simulink model "feedback_linearization_pp_HW_EKF"  (R2023a)
settings: Solver=FixedStepAuto  StartTime=0.0  StopTime=inf  FixedStep=0.001  RelTol=1e-3  EnableMultiTasking=on
values from neighbouring files (symbols this model uses):
  kpp = place(F,G,poles)    [Init_control.m]
  P = 0.5 * eye(6)    [Init_control.m]
undefined symbols (not defined in the file or in its folder): dev, lincontroller, Main, pwm_output0, quadParams
libraries: px4Sensorslib x2, px4lib x1
settings Model: SimulationMode=external  ExtModeTrigDuration=10  Creator=ArriGE66  LastModifiedBy=matte
settings SolverCC: PositivePriorityOrder=on
settings OptimizationCC: EnhancedBackFolding=on  PassReuseOutputArgsAs=Individual arguments  ZeroExternalMemoryAtStartup=off  ZeroInternalMemoryAtStartup=off  MaxStackSize=64  OptimizeBlockOrder=speed  DifferentSizesBufferReuse=on  EfficientTunableParamExpr=on
settings DebuggingCC: ParameterTunabilityLossMsg=error
settings HardwareCC: ProdBitPerPointer=32  ProdBitPerSizeT=32  ProdBitPerPtrDiffT=32  ProdLargestAtomicInteger=Long  ProdLargestAtomicFloat=Double  ProdWordSize=32  ProdLongLongMode=on  ProdHWDeviceType=ARM Compatible->ARM Cortex
settings SFSimCC: MATLABDynamicMemAlloc=off  SimTargetLang=C++
settings RTWCC: Description=Embedded Coder  SystemTargetFile=ert.tlc  HardwareBoard=PX4 Cube Orange  TemplateMakefile=ert_default_tmf  Toolchain=GNU Tools for PX4 Autopilots  TargetLang=C++
settings CodeAppCC: ForceParamTrailComments=on  IgnoreCustomStorageClasses=off  OperatorAnnotations=on  SimulinkDataObjDesc=on  SFDataObjDesc=on  InsertBlockDesc=on
settings ERTTargetCC: ExtMode=on  ExtModeTransport=3  ExtModeStaticAlloc=on  ExtModeStaticAllocSize=1024  ExtModeMexFile=ext_xcp  ExtModeMexArgs=1 COM10 3000000  ExtModeIntrfLevel=Level2 - Open

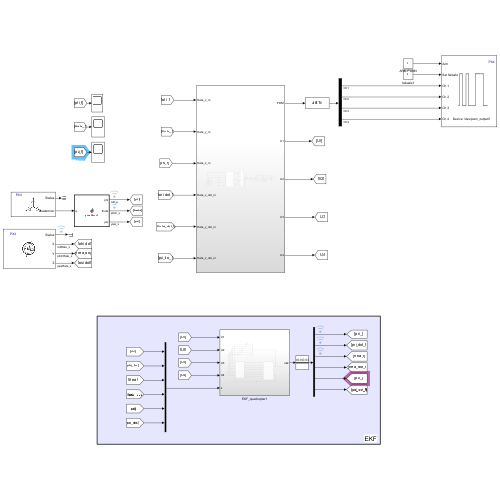
[thumbnail: Simulink's stored preview of the top-level diagram]
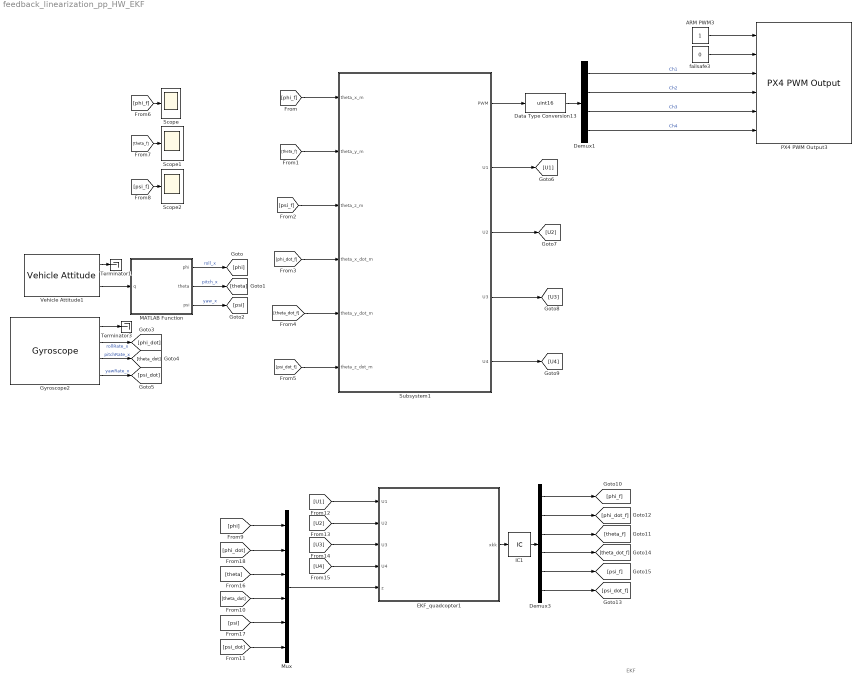
== system feedback_linearization_pp_HW_EKF ==
  note: EKF
  ARM PWM3 : Constant  OutDataTypeStr=boolean  SampleTime=0.002
  Data Type Conversion13 : DataTypeConversion  OutDataTypeStr=uint16  SaturateOnIntegerOverflow=off  RndMeth=Floor
  Demux1 : Demux
  Demux3 : Demux  Outputs=6
  EKF_quadcopter1 : Subsystem
  Gyroscope2 : px4Sensorslib/Gyroscope  uorbTimeStamp=off  BlockingMode=off  BlockTimeout=1e-3  sampleTime=0.002
  IC1 : InitialCondition  Value=[0;0;0;0;0;0]
  MATLAB Function : MATLAB Function  TreatAsAtomicUnit=on
  Mux : Mux  Inputs=6
  PX4 PWM Output3 : px4lib/PX4 PWM Output  pwmDevice=Main (/dev/pwm_output0)  pwmChannel1_=on  pwmChannel2_=on  pwmChannel3_=on  pwmChannel4_=on  pwmChannel5_=off  pwmChannel6_=off  pwmChannel7_=off  pwmChannel8_=off  forceTerminateFailsafe=off  outputErrorStatus=off
  Scope : Scope
  Scope1 : Scope
  Scope2 : Scope
  Subsystem1 : Subsystem
  Terminator1 : Terminator
  Terminator3 : Terminator
  Vehicle Attitude1 : px4Sensorslib/Vehicle Attitude  rollRate=off  pitchRate=off  yawRate=off  quaternion=on  uorbTimeStamp=off  BlockingMode=off  BlockTimeout=0.001  sampleTime=0.002
  failsafe3 : Constant  Value=0  OutDataTypeStr=boolean  SampleTime=0.002
  wires:
  Data Type Conversion13/1 -> Demux1/1
  Demux1/1 -> PX4 PWM Output3/3  "Ch1"
  Demux1/2 -> PX4 PWM Output3/4  "Ch2"
  ARM PWM3/1 -> PX4 PWM Output3/1
  failsafe3/1 -> PX4 PWM Output3/2
  Vehicle Attitude1/2 -> MATLAB Function/1(q)
  Demux1/3 -> PX4 PWM Output3/5  "Ch3"
  Demux1/4 -> PX4 PWM Output3/6  "Ch4"
  Vehicle Attitude1/1 -> Terminator1/1
  Gyroscope2/1 -> Terminator3/1
  Subsystem1/1(PWM) -> Data Type Conversion13/1
  MATLAB Function/1(phi) -> [phi]  "roll_x"
  MATLAB Function/2(theta) -> [theta]  "pitch_x"
  MATLAB Function/3(psi) -> [psi]  "yaw_x"
  Gyroscope2/2 -> [phi_dot]  "rollRate_x"
  Gyroscope2/3 -> [theta_dot]  "pitchRate_x"
  Gyroscope2/4 -> [psi_dot]  "yawRate_x"
  [phi_f] -> Scope/1
  [theta_f] -> Scope1/1
  [psi_f] -> Scope2/1
  [phi_f] -> Subsystem1/1(theta_x_m)
  [psi_f] -> Subsystem1/3(theta_z_m)
  [theta_f] -> Subsystem1/2(theta_y_m)
  [phi_dot_f] -> Subsystem1/4(theta_x_dot_m)
  [theta_dot_f] -> Subsystem1/5(theta_y_dot_m)
  [psi_dot_f] -> Subsystem1/6(theta_z_dot_m)
  [psi_dot] -> Mux/6
  IC1/1 -> Demux3/1
  Demux3/4 -> [theta_dot_f]
  [U4] -> EKF_quadcopter1/4(U4)
  [U2] -> EKF_quadcopter1/2(U2)
  Demux3/3 -> [theta_f]
  [phi_dot] -> Mux/2
  [theta_dot] -> Mux/4
  Demux3/1 -> [phi_f]
  [U1] -> EKF_quadcopter1/1(U1)
  [U3] -> EKF_quadcopter1/3(U3)
  [phi] -> Mux/1
  EKF_quadcopter1/1(xkk) -> IC1/1
  Demux3/2 -> [phi_dot_f]
  Demux3/6 -> [psi_dot_f]
  Demux3/5 -> [psi_f]
  [psi] -> Mux/5
  [theta] -> Mux/3
  Mux/1 -> EKF_quadcopter1/5(z)
  Subsystem1/2(U1) -> [U1]
  Subsystem1/3(U2) -> [U2]
  Subsystem1/4(U3) -> [U3]
  Subsystem1/5(U4) -> [U4]

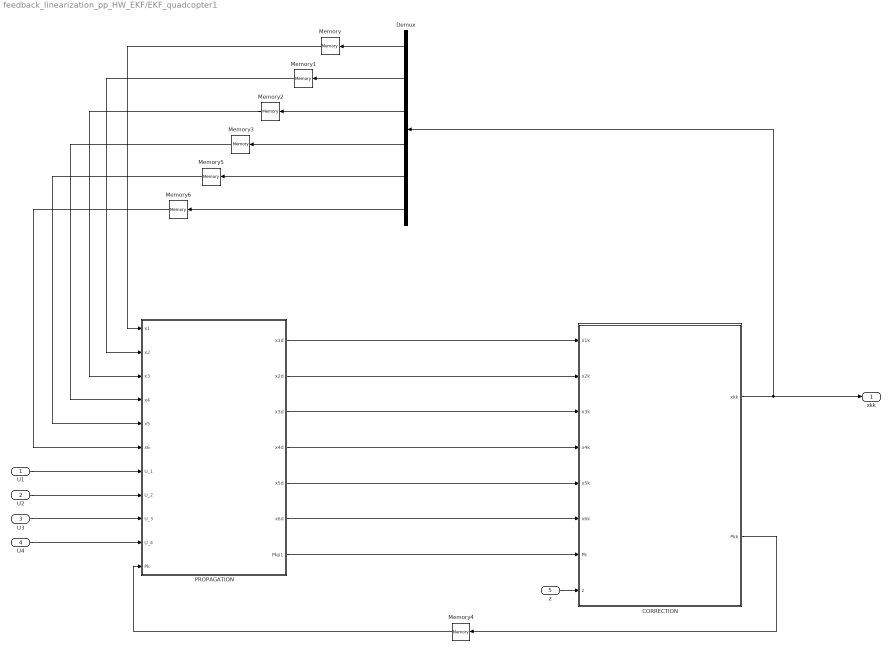
== system feedback_linearization_pp_HW_EKF/EKF_quadcopter1 ==
  U1 : Inport
  U2 : Inport  Port=2
  U3 : Inport  Port=3
  U4 : Inport  Port=4
  z : Inport  Port=5
  CORRECTION : MATLAB Function  TreatAsAtomicUnit=on
  Demux : Demux  Outputs=6
  Memory{,1..3,5..6} (6 alike) : Memory
  Memory4 : Memory  InitialCondition=P
  PROPAGATION : MATLAB Function  TreatAsAtomicUnit=on
  xkk : Outport
  wires:
  PROPAGATION/1(x1d) -> CORRECTION/1(x1k)
  PROPAGATION/2(x2d) -> CORRECTION/2(x2k)
  PROPAGATION/3(x3d) -> CORRECTION/3(x3k)
  PROPAGATION/4(x4d) -> CORRECTION/4(x4k)
  Memory4/1 -> PROPAGATION/11(Pk)
  U1/1 -> PROPAGATION/7(U_1)
  U2/1 -> PROPAGATION/8(U_2)
  U3/1 -> PROPAGATION/9(U_3)
  U4/1 -> PROPAGATION/10(U_4)
  PROPAGATION/7(Pkp1) -> CORRECTION/7(Pk)
  CORRECTION/2(Pkk) -> Memory4/1
  z/1 -> CORRECTION/8(z)
  Demux/1 -> Memory/1
  Demux/2 -> Memory1/1
  Demux/3 -> Memory2/1
  Demux/4 -> Memory3/1
  CORRECTION/1(xkk) -> Demux/1, xkk/1
  Memory/1 -> PROPAGATION/1(x1)
  Memory1/1 -> PROPAGATION/2(x2)
  Memory2/1 -> PROPAGATION/3(x3)
  Memory3/1 -> PROPAGATION/4(x4)
  PROPAGATION/6(x6d) -> CORRECTION/6(x6k)
  PROPAGATION/5(x5d) -> CORRECTION/5(x5k)
  Demux/5 -> Memory5/1
  Memory5/1 -> PROPAGATION/5(x5)
  Demux/6 -> Memory6/1
  Memory6/1 -> PROPAGATION/6(x6)

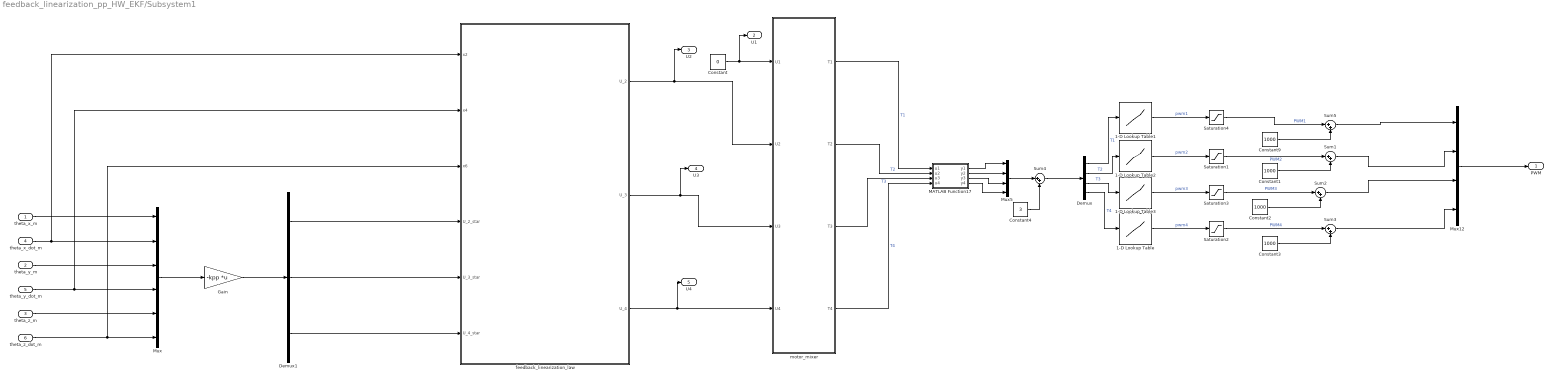
== system feedback_linearization_pp_HW_EKF/Subsystem1 ==
  theta_x_m : Inport
  theta_y_m : Inport  Port=2
  theta_z_m : Inport  Port=3
  theta_x_dot_m : Inport  Port=4
  theta_y_dot_m : Inport  Port=5
  theta_z_dot_m : Inport  Port=6
  1-D Lookup Table : Lookup_n-D  NumberOfTableDimensions=1  BreakpointsForDimension1=[0;0.06477642396;0.16;0.63;2.44;4.43;6.92;8.77;10.52;11.63;12.03;12.09;12.091;12.092;12.093;12.094;12.095;12.096;12.097;12.098;12.099]  Table=[0;50;100;150;200;250;300;350;400;450;500;550;600;650;700;750;800;850;900;950;1000]  InternalRulePriority=Speed  RndMeth=Simplest
  1-D Lookup Table1 : Lookup_n-D  NumberOfTableDimensions=1  BreakpointsForDimension1=[0;0.02;0.06;0.29;0.73;1.07;1.88;2.91;4;5.06;6.71;7.86;9.41;10.86;11.45;11.82;12.07;12.31;12.52;12.74;12.75]  Table=[0;50;100;150;200;250;300;350;400;450;500;550;600;650;700;750;800;850;900;950;1000]  InternalRulePriority=Speed  RndMeth=Simplest
  1-D Lookup Table2 : Lookup_n-D  NumberOfTableDimensions=1  BreakpointsForDimension1=[0;0.05;0.39;1.67;3.19;5.57;8.07;10.01;10.71;11.06;11.42;11.53;11.55;11.551;11.552;11.553;11.554;11.555;11.556;11.557;11.558]  Table=[0;50;100;150;200;250;300;350;400;450;500;550;600;650;700;750;800;850;900;950;1000]  InternalRulePriority=Speed  RndMeth=Simplest
  1-D Lookup Table3 : Lookup_n-D  NumberOfTableDimensions=1  BreakpointsForDimension1=[0;0.06;0.23;0.89;2.47;3.9;5.86;7.81;9.42;10.12;10.6;11.01;11.34;11.39;11.391;11.392;11.393;11.394;11.395;11.396;11.397]  Table=[0;50;100;150;200;250;300;350;400;450;500;550;600;650;700;750;800;850;900;950;1000]  InternalRulePriority=Speed  RndMeth=Simplest
  Constant : Constant  Value=0
  Constant{1..3,9} (4 alike) : Constant  Value=1000  SampleTime=-1
  Constant4 : Constant  Value=3
  Demux : Demux
  Demux1 : Demux  Outputs=3
  Gain : Gain  Gain=-kpp  Multiplication=Matrix(K*u) (u vector)
  MATLAB Function17 : MATLAB Function  TreatAsAtomicUnit=on
  Mux : Mux  Inputs=6
  Mux12 : Mux
  Mux5 : Mux
  Saturation{1..4} (4 alike) : Saturate  UpperLimit=1000  LowerLimit=0
  Sum{1..5} (5 alike) : Sum  Inputs=|++
  feedback_linearization_law : MATLAB Function  TreatAsAtomicUnit=on
  motor_mixer : MATLAB Function  SystemSampleTime=0.004
  PWM : Outport  VectorParamsAs1DForOutWhenUnconnected=off
  U1 : Outport  Port=2
  U2 : Outport  Port=3
  U3 : Outport  Port=4
  U4 : Outport  Port=5
  wires:
  Mux12/1 -> PWM/1
  motor_mixer/4(T4) -> MATLAB Function17/4(u4)  "T4"
  1-D Lookup Table3/1 -> Saturation3/1  "pwm3"
  motor_mixer/1(T1) -> MATLAB Function17/1(u1)  "T1"
  motor_mixer/3(T3) -> MATLAB Function17/3(u3)  "T3"
  1-D Lookup Table2/1 -> Saturation1/1  "pwm2"
  1-D Lookup Table1/1 -> Saturation4/1  "pwm1"
  motor_mixer/2(T2) -> MATLAB Function17/2(u2)  "T2"
  Sum5/1 -> Mux12/1
  Saturation4/1 -> Sum5/1  "PWM1"
  Constant9/1 -> Sum5/2
  1-D Lookup Table/1 -> Saturation2/1  "pwm4"
  Saturation1/1 -> Sum1/1  "PWM2"
  Sum1/1 -> Mux12/2
  Constant1/1 -> Sum1/2
  Saturation3/1 -> Sum2/1  "PWM3"
  Sum2/1 -> Mux12/3
  Constant2/1 -> Sum2/2
  Saturation2/1 -> Sum3/1  "PWM4"
  Sum3/1 -> Mux12/4
  Constant3/1 -> Sum3/2
  Constant4/1 -> Sum4/2
  Demux/3 -> 1-D Lookup Table3/1  "T3"
  Sum4/1 -> Demux/1
  Mux5/1 -> Sum4/1
  MATLAB Function17/3(y3) -> Mux5/3
  MATLAB Function17/1(y1) -> Mux5/1
  MATLAB Function17/4(y4) -> Mux5/4
  Demux/4 -> 1-D Lookup Table/1  "T4"
  MATLAB Function17/2(y2) -> Mux5/2
  Demux/2 -> 1-D Lookup Table2/1  "T2"
  Demux/1 -> 1-D Lookup Table1/1  "T1"
  Constant/1 -> U1/1, motor_mixer/1(U1)
  Demux1/2 -> feedback_linearization_law/5(U_3_star)
  theta_y_m/1 -> Mux/3
  Demux1/3 -> feedback_linearization_law/6(U_4_star)
  theta_z_dot_m/1 -> feedback_linearization_law/3(x6), Mux/6
  theta_z_m/1 -> Mux/5
  theta_y_dot_m/1 -> feedback_linearization_law/2(x4), Mux/4
  Mux/1 -> Gain/1
  Demux1/1 -> feedback_linearization_law/4(U_2_star)
  theta_x_dot_m/1 -> feedback_linearization_law/1(x2), Mux/2
  theta_x_m/1 -> Mux/1
  Gain/1 -> Demux1/1
  feedback_linearization_law/1(U_2) -> U2/1, motor_mixer/2(U2)
  feedback_linearization_law/2(U_3) -> U3/1, motor_mixer/3(U3)
  feedback_linearization_law/3(U_4) -> U4/1, motor_mixer/4(U4)

== matlab function feedback_linearization_pp_HW_EKF/Subsystem1/motor_mixer ==
  data: U1 input; T1 output; U2 input; U3 input; U4 input; T2 output; T3 output; T4 output; quadParams parameter
function [T1,T2,T3,T4] = motor_mixer(U1,U2,U3,U4,quadParams)
%Function description:
%  Control allocation. The quadrotor type is X-configuration,
%  and the airframe is as follows:
%3↓   1↑
 %  \ /
 %  / \
 %2↑   4↓


% |U1|    |       1             1           1            1       |  |T1|
% |U2|  = | -L*sqrt(2)/2  L*sqrt(2)/2  L*sqrt(2)/2  -L*sqrt(2)/2 |  |T2|
% |U3|    | L*sqrt(2)/2  -L*sqrt(2)/2  L*sqrt(2)/2  -L*sqrt(2)/2 |  |T3| 
% |U4|    | kd/kt            kd/kt       -kd/kt       -kd/kt     |  |T4|



% we need to invert this in order to obtain 
% |T1|                              |U1|
% |T2| =  quadParams.MotorMixer *   |U2|
% |T3|                              |U3|
% |T4|                              |U4|

U=[U1;U2;U3;U4];
T=quadParams.MotorMixer*U;
T1=T(1);
T2=T(2);
T3=T(3);
T4=T(4);

== matlab function feedback_linearization_pp_HW_EKF/EKF_quadcopter1/CORRECTION ==
  data: x1k input; xkk output; Pkk output; x2k input; x3k input; x4k input; x5k input; x6k input; Pk input; z input
function [xkk,Pkk] = fcn(x1k,x2k,x3k,x4k,x5k,x6k,Pk,z)

% R = [2.782739102258347e-06 0 0 0 0 0;
%      0 1.936548166270313e-08 0 0 0 0;
%      0 0 2.718240466492716e-06 0 0 0;
%      0 0 0 1.809123162388460e-08 0 0;
%      0 0 0 0 5.587443411059212e-06 0;
%      0 0 0 0 0 5.587443411059212e-06];

R = [1.936548166270313e-08 0 0 0 0 0;
     0 2.782739102258347e-06 0 0 0 0;
     0 0 1.809123162388460e-08 0 0 0;
     0 0 0 2.718240466492716e-06 0 0;
     0 0 0 0 5.587443411059212e-06 0;
     0 0 0 0 0 2.976654513986432e-06];

H = [1 0 0 0 0 0;
     0 1 0 0 0 0;
     0 0 1 0 0 0;
     0 0 0 1 0 0;
     0 0 0 0 1 0;
     0 0 0 0 0 1];

xk = [x1k;x2k;x3k;x4k;x5k;x6k];

y = z - H * xk;

K = Pk*(H')/(H*Pk*(H') + R);

xkk = xk + K * y;
Pkk = (eye(6)-K * H) * Pk;

== matlab function feedback_linearization_pp_HW_EKF/EKF_quadcopter1/PROPAGATION ==
  data: x1 input; x1d output; x2 input; x3 input; x4 input; x5 input; x6 input; U_1 input; U_2 input; U_3 input; U_4 input; x2d output; x3d output; x4d output; x5d output; x6d output; Pk input; Pkp1 output
function [x1d,x2d,x3d,x4d,x5d,x6d,Pkp1] = fcn(x1,x2,x3,x4,x5,x6,U_1,U_2,U_3,U_4,Pk)

quadParams.g = 9.81;
quadParams.m = 1.07;
quadParams.Jx = 0.055;
quadParams.Jy = 0.055;
quadParams.Jz = 0.03;
quadParams.Jr=0;
quadParams.d = 0.1;
quadParams.L = 0.25;
quadParams.kd= 1.779e-07;  %Rotor torque coefficient(kg.m^2)   %M=kd*w^2
quadParams.kt = 1.105e-05;  %Rotor thrust coefficient(kg.m^2)  %T=kt*w^2

m = 1.07;
L = 0.25;
d = 0.055;
J = 0.055;
g = 9.81;
Ts = 0.002;

% Q = [0.0000000001 0 0 0 0 0;
%      0 0.00000001 0 0 0 0;
%      0 0 0.0000000001 0 0 0;
%      0 0 0 0.00000001 0 0;
%      0 0 0 0 0.0000000001 0;
%      0 0 0 0 0 0.00000001];

Q = [5e-16 0 0 0 0 0;
     0 1e-6 0 0 0 0;
     0 0 5e-16 0  0 0;
     0 0 0 1e-6 0 0;
     0 0 0 0 1e-13 0;
     0 0 0 0 0 5e-7];


a1=(quadParams.Jy-quadParams.Jz)/quadParams.Jx;
a2=-quadParams.Jr/quadParams.Jx;
a3=(quadParams.Jz-quadParams.Jx)/quadParams.Jy;
a4=quadParams.Jr/quadParams.Jy;
a5=(quadParams.Jx-quadParams.Jy)/quadParams.Jz;
b1=quadParams.L/quadParams.Jx;
b2=quadParams.L/quadParams.Jy;
b3=quadParams.L/quadParams.Jz;


x1d_dot =x2;

x2d_dot =x4*x6*a1 + b1*U_2;

x3d_dot =x4;

x4d_dot =x2*x6*a3+b2*U_3;

x5d_dot =x6;

x6d_dot =x4*x2*a5+b3*U_4;

x1d = x1 + x1d_dot*Ts;
x2d = x2 + x2d_dot*Ts;
x3d = x3 + x3d_dot*Ts;
x4d = x4 + x4d_dot*Ts;
x5d = x5 + x5d_dot*Ts;
x6d = x6 + x6d_dot*Ts;


F11 = 0;
F12 = 1;
F13 = 0;
F14 = 0;
F15 = 0;
F16 = 0;

F21 = 0;
F22 = 0;
F23 = 0;
F24 = x6*a1;
F25 = 0;
F26 = x4*a1;

F31 = 0;
F32 = 0;
F33 = 0;
F34 = 1;
F35 = 0;
F36 = 0;

F41 = 0;
F42 = x6*a3;
F43 = 0;
F44 = 0;
F45 = 0;
F46 = x2*a3;

F51 = 0;
F52 = 0;
F53 = 0;
F54 = 0;
F55 = 0;
F56 = 1;

F61 = 0;
F62 = x4*a5;
F63 = 0;
F64 = x2*a5;
F65 = 0;
F66 = 0;

F = [F11 F12 F13 F14 F15 F16;
     F21 F22 F23 F24 F25 F26;
     F31 F32 F33 F34 F35 F36;
     F41 F42 F43 F44 F45 F46;
     F51 F52 F53 F54 F55 F56;
     F61 F62 F63 F64 F65 F66];

PHI = expm(F * Ts);

Pkp1 = PHI * Pk * (PHI') + Q;

== matlab function feedback_linearization_pp_HW_EKF/MATLAB Function ==
  data: q input; phi output; theta output; psi output
function [phi,theta,psi] = quat2eul(q)
% Conversion from Quaternion to Euler angles based on the PX4 Firmware
% v1.6.5 release.
% 
% Quaternion -> DCM -> Euler Angles
% INPUT:
%   q: Quaternion vector of the format: (a + bi + cj + dk)
% OUTPUT:
%   [phi,theta,psi]: Euler angles in radians.
% 
 
    a = q(1);
    b = q(2);
    c = q(3);
    d = q(4);

    aSq = a*a;
    bSq = b*b;
    cSq = c*c;
    dSq = d*d;

    d_pi2 = pi/2;

    % quaternion_to_dcm
    dcm00 = aSq + bSq - cSq - dSq;
    % dcm01 = 2*(b*c - a*d);
    dcm02 = 2*(a*c + b*d);
    dcm10 = 2*(b*c + a*d);
    % dcm11 = aSq - bSq + cSq - dSq;
    dcm12 = 2*(c*d - a*b);
    dcm20 = 2*(b*d - a*c);
    dcm21 = 2*(a*b + c*d);
    dcm22 = aSq - bSq - cSq + dSq;

    % dcm_to_euler
    theta = asin(-dcm20);
    if abs(theta - d_pi2) < 1.0e-3
        phi = single(0.0);
        psi = atan2(dcm12, dcm02);
    elseif abs(theta + d_pi2) < 1.0e-3
        phi = single(0.0);
        psi = atan2(-dcm12, -dcm02);
    else
        phi = atan2(dcm21, dcm22);
        psi = atan2(dcm10, dcm00);
    end

end

== matlab function feedback_linearization_pp_HW_EKF/Subsystem1/MATLAB Function17 ==
  data: u1 input; y1 output; u2 input; u3 input; u4 input; y2 output; y3 output; y4 output
function [y1,y2,y3,y4] = fcn(u1,u2,u3,u4)

if u1 < 0
    u2 = u2 + abs(u1);
    u1 = u1+abs(u1);
end
if u2 < 0
    u2 = u2 + abs(u2);
    u1 = u1 + abs(u2);
end
if u3 < 0
    u3 = u3 + abs(u3);
    u4 = u4 + abs(u3);
end    
if u4 < 0
    u4 = u4 + abs(u4);
    u3 = u3 + abs(u4);
end
 y1 = u1;
 y2 = u2;
 y3 = u3;
 y4 = u4;

== matlab function feedback_linearization_pp_HW_EKF/Subsystem1/feedback_linearization_law ==
  data: x2 input; x4 input; x6 input; U_2_star input; U_2 output; U_3_star input; U_4_star input; U_3 output; U_4 output; lincontroller parameter; quadParams parameter
function [U_2,U_3,U_4] = feedback_linearization_law(x2,x4,x6,U_2_star,U_3_star,U_4_star,lincontroller,quadParams)


a1=(quadParams.Jy-quadParams.Jz)/quadParams.Jx;
a2=-quadParams.Jr/quadParams.Jx;
a3=(quadParams.Jz-quadParams.Jx)/quadParams.Jy;
a4=quadParams.Jr/quadParams.Jy;
a5=(quadParams.Jx-quadParams.Jy)/quadParams.Jz;
b1=quadParams.L/quadParams.Jx;
b2=quadParams.L/quadParams.Jy;
b3=quadParams.L/quadParams.Jz;



f_2 = 1/b1*(lincontroller.K2*x2-x4*x6*a1);
f_3 = 1/b2*(lincontroller.K3*x4-x2*x6*a3);
f_4 = 1/b3*(lincontroller.K4*x6-x4*x2*a5);


U_2 = f_2 + U_2_star;
U_3 = f_3 + U_3_star;
U_4 = f_4 + U_4_star;
